simulink model "Cruise_control_Plant"  (R2020b)
settings: Solver=VariableStepAuto  StartTime=0.0  StopTime=120  RelTol=1e-3
undefined symbols (not defined in the file): b, m
settings Model: DataDictionary=Data_Dictionary_for_Variables.sldd  Creator=intel  LastModifiedBy=intel
settings DataIOCC: SaveOutput=off  SaveTime=off

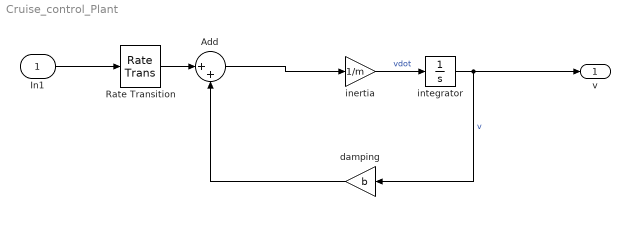
== system Cruise_control_Plant ==
  In1 : Inport  OutDataTypeStr=double  PortDimensions=1  SampleTime=[0,1]
  Add : Sum  Inputs=|++
  Rate Transition : RateTransition
  damping : Gain  Gain=b
  inertia : Gain  Gain=1/m
  integrator : Integrator
  v : Outport  OutDataTypeStr=double  PortDimensions=1  SampleTime=0
  wires:
  Add/1 -> inertia/1
  integrator/1 -> damping/1, v/1  "v"
  damping/1 -> Add/2
  inertia/1 -> integrator/1  "vdot"
  Rate Transition/1 -> Add/1
  In1/1 -> Rate Transition/1
